simulink model "scheme_fullbodycontrol"  (R2025a)
settings: Solver=ode3  StartTime=0.0  StopTime=40  FixedStep=dt  RelTol=1e-3
values from neighbouring files (symbols this model uses):
  dt = 0.0005    [Planning_Sim.m]
  goal_pos = waypoints(end, :)'    [Planning_Sim.m]
  initial_positions_rad = rawJointPositions(1, :)'    [manipulator_sim.m]
  manipulator_position_data = positions_final    [manipulator_sim.m]
  manipulator_time_vector = time_final    [manipulator_sim.m]
  op_space_pose_trajectory = zeros(4, 4, num_points)    [Planning_Sim.m]
  waypoints = pathObj.States(:, 1:2)    [Planning_Sim.m]
  x0 = zeros(14, 1)    [Planning_Sim.m]
undefined symbols (not defined in the file or in its folder): control_params, p, X, Y, Z
libraries: sm_lib x186, nesl_utility x34, fl_lib x3
(part 5 of 5)

== matlab function scheme_fullbodycontrol/BallBot Plant1/MATLAB Function ==
  data: dx output; x input; p parameter; tau input; wrench_ext input
function dx = stateDerivative3D_with_exforce(x, p, tau, wrench_ext)
    % MODIFICATION 1: The function now accepts a 4th argument, 'wrench_ext',
    % which is a vector containing the external forces and torques from Simulink.
    
    % Unpack state vector (10 elements)
    theta_x = x(1); dot_theta_x = x(6);
    theta_y = x(2); dot_theta_y = x(7);
    theta_z = x(3); dot_theta_z = x(8);
    % phi_x   = x(4); % Not needed for dynamics
    % phi_y   = x(5); % Not needed for dynamics
    dot_phi_x   = x(9);
    dot_phi_y   = x(10);
    
    % Unpack input torques
    tau_x = tau(1);
    tau_y = tau(2);
    tau_z = tau(3);

     % Unpack the external wrench vector from the new input ---
    % Expected order: [F_px, F_py, F_pz, tau_px, tau_py]
    F_px   = wrench_ext(1);
    F_py   = wrench_ext(2);
    F_pz   = wrench_ext(3);
    tau_px = wrench_ext(4);
    tau_py = wrench_ext(5);

    % --- Prepare arguments for auto-generated functions ---
    % Create separate parameter vectors for each plane, now including h_app
    % Note: I_Ux is for roll, I_Uy is for pitch.
    params_arg_roll = [p.m_U,  p.I_Uy, p.I_Ux, p.l_U, p.m_S, p.I_S, p.r_S, p.g, p.h_app, p.b_theta, p.b_phi];
    params_arg_pitch = [p.m_U, p.I_Uy, p.I_Ux, p.l_U, p.m_S, p.I_S, p.r_S, p.g,p.h_app, p.b_theta, p.b_phi];
    
    external_vars_x = [F_py, F_pz, tau_px]; % For Roll dynamics
    external_vars_y = [F_px, F_pz, tau_py]; % For Pitch dynamics

    % --- X-Z Plane (Roll) Dynamics ---
    states_arg_x = [theta_x, dot_theta_x, dot_phi_x];
    inputs_arg_x = [tau_x];
    ddot_theta_x = copy_autogen_ddot_theta_x(states_arg_x, inputs_arg_x, params_arg_roll, external_vars_x);
    ddot_phi_x   = copy_autogen_ddot_phi_x(states_arg_x, inputs_arg_x, params_arg_roll, external_vars_x);
    

    % --- Y-Z Plane (Pitch) Dynamics ---
    states_arg_y = [theta_y, dot_theta_y, dot_phi_y];
    inputs_arg_y = [tau_y];
    ddot_theta_y = copy_autogen_ddot_theta_y(states_arg_y, inputs_arg_y, params_arg_pitch, external_vars_y);
    ddot_phi_y   = copy_autogen_ddot_phi_y(states_arg_y, inputs_arg_y, params_arg_pitch, external_vars_y);
    
    % --- Transversal Plane Dynamics (Yaw) ---
    % external forces at the center of the top surface are assumed not to produce yaw torque.
    ddot_theta_z = (tau_z - p.fz * dot_theta_z) / p.Iz;
    
    % --- Assemble the state derivative vector dx ---
    dx = [
        dot_theta_x;    % dx(1) = d(theta_x)/dt
        dot_theta_y;    % dx(2) = d(theta_y)/dt
        dot_theta_z;    % dx(3) = d(theta_z)/dt
        dot_phi_x;      % dx(4) = d(phi_x)/dt
        dot_phi_y;      % dx(5) = d(phi_y)/dt
        ddot_theta_x;   % dx(6) = d(dot_theta_x)/dt
        ddot_theta_y;   % dx(7) = d(dot_theta_y)/dt
        ddot_theta_z;   % dx(8) = d(dot_theta_z)/dt
        ddot_phi_x;     % dx(9) = d(dot_phi_x)/dt
        ddot_phi_y;     % dx(10)= d(dot_phi_y)/dt
    ];
end

== matlab function scheme_fullbodycontrol/MATLAB Function ==
  settings: updateMethod=DISCRETE
  data: x input; phi_dot_c output; waypoints input; p parameter; simtime input; control_params parameter; is_final_segment output; dt parameter
function [phi_dot_c, is_final_segment] = generate_ff_fb_velocity_command(x,waypoints, p, simtime, control_params, dt)
% =========================================================================
% ADVANCED FEEDFORWARD + FEEDBACK VELOCITY COMMAND GENERATOR
%
% Version: 5.1 - NO REPLANNING (Plan Once, Execute)
% This is the complete, self-contained version with all helper functions.
% =========================================================================

% --- Parameters ---
persistent processed_path;
persistent integral_pos_error; % NEW: Persistent variable for the integral term

v_max       = 0.3;
a_max       = 0.08;
Kp_feedback = 0.20; % Gain for path following on intermediate segments
lookahead_distance = 0.0;
Kp_final_approach = control_params.Kp;
Ki_final_approach = control_params.Ki; % Get the new Ki gain from your main script

% --- Current Robot State ---
p_current = [p.r_S * x(5); -p.r_S * x(4)];
v_current = [p.r_S * x(2); -p.r_S * x(3)];

% --- PLAN-ONCE LOGIC ---
% This block will only run ONCE for the entire simulation.
if isempty(processed_path)
    disp('Initial (and only) path processing...');
    processed_path = preprocess_waypoints_with_blending(waypoints, v_max, a_max, ...
                                                        p_current, v_current, simtime);
end

% --- Hybrid Control Logic ---
[v_ref_normal, ~, segment_is_valid, current_segment_idx] = get_reference_and_segment(processed_path, simtime);

if isempty(processed_path)
    num_total_segments = 0;
else
    num_total_segments = length(processed_path.segments);
end

if isempty(integral_pos_error)
    integral_pos_error = zeros(2,1);
end

is_final_segment = (segment_is_valid && current_segment_idx == num_total_segments);

if is_final_segment
    % Final Approach: Regulation Controller
    p_goal = waypoints(end, :)';
    position_error = p_goal - p_current;
   integral_pos_error = integral_pos_error + position_error * dt;
    v_cmd = Kp_final_approach * position_error + Ki_final_approach * integral_pos_error;

else
    if(1)
        % Path Following: Advanced Controller (using a fixed target for simplicity)
        % You can re-integrate the full lookahead logic here if needed.
        p_target_for_feedback = waypoints(min(current_segment_idx + 1, size(waypoints,1)), :)';

    else
        % --- Inizio Logica Lookahead ---
        % 1. Proietta la posizione corrente del robot sul segmento di percorso attuale.
        current_segment = processed_path.segments(current_segment_idx);
        vec_to_robot = p_current - current_segment.p_start;
        proj_dist_on_segment = dot(vec_to_robot, current_segment.direction);
        proj_dist_on_segment = max(0, min(current_segment.distance, proj_dist_on_segment)); % Limita la proiezione al segmento
        integral_pos_error = zeros(2,1);

        % 2. Inizia la ricerca del punto di lookahead dalla proiezione del robot.
        dist_to_travel = lookahead_distance;
        p_target_for_feedback = current_segment.p_start + proj_dist_on_segment * current_segment.direction;
        
        % 3. "Avanza" lungo il percorso della distanza di lookahead, saltando tra i segmenti se necessario.
        for i = current_segment_idx:num_total_segments
            segment_i = processed_path.segments(i);
            
            % Calcola la distanza rimanente sul segmento corrente (o la lunghezza totale per i successivi).
            if i == current_segment_idx
                dist_left_on_segment = segment_i.distance - proj_dist_on_segment;
            else
                dist_left_on_segment = segment_i.distance;
            end
            
            if dist_to_travel <= dist_left_on_segment
                % Il punto target si trova su questo segmento.
                p_target_for_feedback = p_target_for_feedback + dist_to_travel * segment_i.direction;
                break; % Esci dal ciclo una volta trovato il punto.
            else
                % Il punto target è oltre questo segmento. Salta alla fine di questo segmento
                % e riduci la distanza ancora da percorrere.
                dist_to_travel = dist_to_travel - dist_left_on_segment;
                p_target_for_feedback = segment_i.p_end;
            end
        end
        % --- Fine Logica Lookahead ---
    end
    position_error = p_target_for_feedback - p_current;
    v_feedback = Kp_feedback * position_error;
    v_cmd = v_ref_normal + v_feedback;
end

    % --- Initialization Override ---
    initialization_time = 3.0;
    if simtime < initialization_time
        position_error_init = [0;0] - p_current;
        v_cmd = Kp_final_approach * position_error_init;
    end

    % --- Final Command Generation ---
    v_cmd_magnitude = norm(v_cmd);
    if v_cmd_magnitude > v_max
        v_cmd = v_cmd / v_cmd_magnitude * v_max;
    end
    phi_dot_c = [v_cmd(1) / p.r_S; -v_cmd(2) / p.r_S];
end

% =========================================================================
% --- LOCAL HELPER FUNCTIONS (MUST BE IN THE SAME FILE) ---
% =========================================================================
function processed_path = preprocess_waypoints_with_blending(waypoints, v_max, a_max, p_start_robot, v_start_robot, time_start_robot)
    effective_waypoints = [p_start_robot'; waypoints];
    num_waypoints = size(effective_waypoints, 1);
    num_segments = num_waypoints - 1;
    
    segment_template = struct('p_start', zeros(2,1), 'p_end', zeros(2,1), 'distance', 0, 'direction', zeros(2,1));
    path_geom.segments = repmat(segment_template, 1, num_segments);
    for i = 1:num_segments
        p_start = effective_waypoints(i, :)';
        p_end   = effective_waypoints(i+1, :)';
        vec     = p_end - p_start;
        dist    = norm(vec);
        path_geom.segments(i).p_start   = p_start;
        path_geom.segments(i).p_end     = p_end;
        path_geom.segments(i).distance  = dist;
        if dist > 1e-6
            path_geom.segments(i).direction = vec / dist;
        else
            path_geom.segments(i).direction = zeros(2,1);
        end
    end
    
    v_transitions = zeros(2, num_waypoints);
    v_transitions(:, 1) = v_start_robot;
    v_transitions(:, end) = [0; 0];
    alpha = 1.0;
    
    for i = 2:num_waypoints-1
        v_max_for_corner = v_max;
        if i >= num_waypoints - 2 
            v_max_for_corner = v_max / 2;
        end
        dir_in  = path_geom.segments(i-1).direction;
        dir_out = path_geom.segments(i).direction;
        cos_theta = dot(dir_in, dir_out);

        % CALCOLO CHIAVE: La magnitudine della velocità all'angolo.
        % Se i segmenti sono dritti (cos_theta=1), v_mag = v_max.
        % Se l'angolo è di 90° (cos_theta=0), v_mag = 0.5 * v_max.
        % Se è un tornante (cos_theta=-1), v_mag = 0.
        v_mag = v_max_for_corner * ((1 + cos_theta) / 2)^alpha;

        % CALCOLO CHIAVE: La direzione della velocità all'angolo.
        % La somma dei due versori dà un vettore che biseca l'angolo,
        % che è la direzione ottimale per attraversare la curva.
        v_dir_vec = dir_in + dir_out;

        if norm(v_dir_vec) > 1e-6
            v_dir_normalized = v_dir_vec / norm(v_dir_vec);
        else
            v_dir_normalized = zeros(2,1);
            v_mag = 0;
        end
        v_transitions(:, i) = v_mag * v_dir_normalized;
    end
    
    % Calcolate le informazioni geometriche e le velocità di transizione,
    % costruisce un profilo di velocità temporale
    profile_template = struct('v_start',0,'v_cruise',0,'v_end',0,'t_accel',0,'t_const',0,'t_decel',0,'total_time',0,'start_time',0,'a_max',0);
    processed_segment_template = struct('profile',profile_template,'direction',zeros(2,1),'p_start',zeros(2,1),'p_end',zeros(2,1),'distance',0);
    processed_segments = repmat(processed_segment_template, 1, num_segments);
    
    cumulative_time = time_start_robot;
    for i = 1:num_segments
        v_max_current = v_max;
        a_max_current = a_max;
        % Rallenta la velocità e l'accelerazione per gli ultimi segmenti.
        if i >= num_segments - 1 && num_segments > 1
            v_max_current = v_max / 2;
            a_max_current = a_max / 2;
        elseif num_segments == 1
             v_max_current = v_max / 2;
             a_max_current = a_max / 2;
        end
        segment = path_geom.segments(i);

        % Proietta i VETTORI velocità di transizione sulla DIREZIONE del segmento attuale.
        % Questo ci dà la velocità SCALARE di inizio e fine LUNGO il segmento.
        v_start = dot(v_transitions(:, i),   segment.direction);
        v_end   = dot(v_transitions(:, i+1), segment.direction);
        v_start = max(0, v_start);
        v_end   = max(0, v_end);
        
         % Usa le equazioni cinematiche per calcolare la distanza necessaria per
        % accelerare e decelerare tra v_start, v_end e la v_max del segmento.
        dist_accel = (v_max_current^2 - v_start^2) / (2 * a_max_current);
        dist_decel = (v_max_current^2 - v_end^2)   / (2 * a_max_current);

        % Controlla se il segmento è abbastanza lungo per raggiungere la velocità massima.
        if (dist_accel + dist_decel) >= segment.distance
            % NO: Profilo TRIANGOLARE. Il robot non raggiunge v_max.
            % Calcola la velocità di picco (v_cruise) che può raggiungere.
            v_peak_sq = (2*a_max_current*segment.distance + v_start^2 + v_end^2) / 2;
            v_cruise = sqrt(max(0, v_peak_sq));
            t_accel = (v_cruise - v_start) / a_max_current;
            t_const = 0;
            t_decel = (v_cruise - v_end) / a_max_current;
        else
            % SÌ: Profilo TRAPEZOIDALE. Il robot raggiunge v_max.
            v_cruise = v_max_current;
            dist_const = segment.distance - dist_accel - dist_decel;
            t_accel = (v_cruise - v_start) / a_max_current;
            t_const = dist_const / v_cruise;
            t_decel = (v_cruise - v_end) / a_max_current;
        end
        % Salva tutti i dati calcolati..
        processed_segments(i).profile.v_start  = v_start;
        processed_segments(i).profile.v_cruise = v_cruise;
        processed_segments(i).profile.v_end    = v_end;
        processed_segments(i).profile.t_accel  = max(0, t_accel);
        processed_segments(i).profile.t_const  = max(0, t_const);
        processed_segments(i).profile.t_decel  = max(0, t_decel);
        processed_segments(i).profile.total_time = processed_segments(i).profile.t_accel + processed_segments(i).profile.t_const + processed_segments(i).profile.t_decel;
        processed_segments(i).profile.start_time = cumulative_time;
        processed_segments(i).profile.a_max = a_max_current;
        
        processed_segments(i).direction = segment.direction;
        processed_segments(i).p_start = segment.p_start;
        processed_segments(i).p_end = segment.p_end;
        processed_segments(i).distance = segment.distance;
        
        cumulative_time = cumulative_time + processed_segments(i).profile.total_time;
    end
    processed_path.segments = processed_segments;
    processed_path.total_duration = cumulative_time;
end
% -------------------------------------------------------------------------
function [v_ref, segment, is_valid, current_segment_idx] = get_reference_and_segment(processed_path, simtime)
    profile_template = struct('v_start',0,'v_cruise',0,'v_end',0,'t_accel',0,'t_const',0,'t_decel',0,'total_time',0,'start_time',0,'a_max',0);
    segment_template = struct('profile',profile_template,'direction',zeros(2,1),'p_start',zeros(2,1),'p_end',zeros(2,1),'distance',0);
    
    segment = segment_template; 
    v_ref = [0;0];
    is_valid = false;
    current_segment_idx = 0; 
    
    if ~isempty(processed_path) && ~isempty(processed_path.segments)
        for i = 1:length(processed_path.segments)
            if simtime >= processed_path.segments(i).profile.start_time
                current_segment_idx = i;
            else
                break;
            end
        end
        segment = processed_path.segments(current_segment_idx);
        is_valid = true;
        prof = segment.profile;
        a_max_current = prof.a_max; 
        
        if simtime >= processed_path.total_duration
            v_ref = [0; 0];
            return;
        end
        time_in_segment = simtime - prof.start_time;
        current_speed = 0.0;
        
        if time_in_segment < prof.t_accel
            current_speed = prof.v_start + a_max_current * time_in_segment;
        elseif time_in_segment < (prof.t_accel + prof.t_const)
            current_speed = prof.v_cruise;
        else
            time_in_decel = time_in_segment - (prof.t_accel + prof.t_const);
            current_speed = prof.v_cruise - a_max_current * time_in_decel;
        end
        v_ref = max(0, current_speed) * segment.direction;
    end
end

== matlab function scheme_fullbodycontrol/MATLAB Function1 ==
  settings: updateMethod=DISCRETE
  data: alpha_traj input; thetaz_des output; thetaz input; external_wrench input
function thetaz_des = calculate_desired_yaw(alpha_traj, thetaz, external_wrench)
% =========================================================================
% CALCULATE DESIRED YAW (v3.0 - With Continuous Unwrapping)
%
% This version removes the final normalization and implements an unwrapping
% algorithm. This allows the desired yaw angle to grow continuously beyond
% +/- 180 degrees, enabling smooth, continuous rotation without wrapping.
% =========================================================================

    % --- NEW: Persistent variable to store the last output for unwrapping ---
    persistent thetaz_des_old;
    if isempty(thetaz_des_old)
        % Initialize to the robot's starting yaw angle on the first run
        thetaz_des_old = thetaz;
    end

    % --- Step 1 & 2: Calculate instantaneous desired angle (Unchanged) ---
    F_dist_world_x = external_wrench(1);
    F_dist_world_y = external_wrench(2);
    local_psi_des = 0.0;
    force_magnitude = sqrt(F_dist_world_x^2 + F_dist_world_y^2);
    
    if force_magnitude < 1e-6
        local_psi_des = alpha_traj;
    else
        c = cos(-thetaz);
        s = sin(-thetaz);
        F_dist_body_x = c * F_dist_world_x - s * F_dist_world_y;
        F_dist_body_y = s * F_dist_world_x + c * F_dist_world_y;
        beta_dist_body = atan2(F_dist_body_y, F_dist_body_x);
        local_psi_des = alpha_traj - beta_dist_body;
    end
    
    % --- Step 3: UNWRAP the angle for continuous rotation ---
    % Instead of normalizing the final value, we normalize the DIFFERENCE
    % between the new instantaneous angle and the last continuous angle.
    
    angle_diff = local_psi_des - thetaz_des_old;
    
    % Find the shortest rotation path (wrap the difference to [-pi, pi])
    angle_diff_wrapped = atan2(sin(angle_diff), cos(angle_diff));
    
    % Add this shortest-path difference to the previous angle to get the
    % new continuous, unwrapped angle.
    thetaz_des = thetaz_des_old + angle_diff_wrapped;
    
    % --- Step 4: Update the persistent variable for the next time step ---
    thetaz_des_old = thetaz_des;

end

== matlab function scheme_fullbodycontrol/Smart LookUpTable ==
  settings: updateMethod=DISCRETE
  data: T_desired output; EUL output; t_in input; op_space_pose_trajectory parameter; manipulator_time_vector parameter; P output
function [T_desired, EUL, P] = get_pose_from_trajectory(t_in, op_space_pose_trajectory, manipulator_time_vector)
% =========================================================================
% TRAJECTORY INTERPOLATOR AND POSE SPLITTER (v4.1 - Column Vector Fix)
%
% This version transposes the EUL output to be a column vector [3x1]
% to match the expectation of downstream Simulink blocks like Demux.
% =========================================================================
    % For Coder compatibility, explicitly define the output sizes.
    P = zeros(3, 1);
    % FIX 1: Initialize EUL as a 3x1 column vector.
    EUL = zeros(3, 1);
    T_desired = eye(4);
    % Use a persistent variable to show warnings only once per simulation.
    persistent has_warned;
    if isempty(has_warned)
        has_warned = false;
    end

    % --- 1. Input Sanity Checks ---
    if isnan(t_in)
        if ~has_warned
            warning('Input time t_in is NaN. Outputting a zero pose.');
            has_warned = true;
        end
        return; % Exit with P and EUL as zeros
    end
    
    if isempty(manipulator_time_vector) || isempty(op_space_pose_trajectory)
        if ~has_warned
            warning('Trajectory data is empty. Outputting a zero pose.');
            has_warned = true;
        end
        return; % Exit with P and EUL as zeros
    end

    % --- 2. Data Formatting ---
    if isrow(manipulator_time_vector)
        manipulator_time_vector = manipulator_time_vector';
    end

    % --- 3. Interpolation ---
    if isscalar(manipulator_time_vector)
        T_interpolated = op_space_pose_trajectory(:,:,1);
    else
        num_points = size(op_space_pose_trajectory, 3);
        data_reshaped = reshape(op_space_pose_trajectory, 16, num_points)';
        
        interpolated_row = interp1(manipulator_time_vector, data_reshaped, t_in, 'linear', 'extrap');
        
        if any(isnan(interpolated_row))
             if ~has_warned
                warning('Interpolation resulted in NaN. Holding first pose as fallback.');
                has_warned = true;
             end
             T_interpolated = op_space_pose_trajectory(:,:,1);
        else
             T_interpolated = reshape(interpolated_row, 4, 4);
        end
    end
    
    % --- 4. Split the Result into Position and Euler Angles ---
    P = T_interpolated(1:3, 4);
    R = T_interpolated(1:3, 1:3);
    T_desired = T_interpolated;
    
    % FIX 2: Transpose the output of rotm2eul to create a column vector.
    EUL = rotm2eul(R, 'ZYX')'; % <-- The fix is the transpose operator '

end
